simulink model "Gesha1slmodif"  (R2022b)
settings: Solver=VariableStepAuto  StartTime=0.0  StopTime=10.0  RelTol=1e-3
undefined symbols (not defined in the file or in its folder): DiscIntNeverNeededParam
libraries: simulink x13, rllib x1
settings Model: Creator=yonat  LastModifiedBy=Gesha

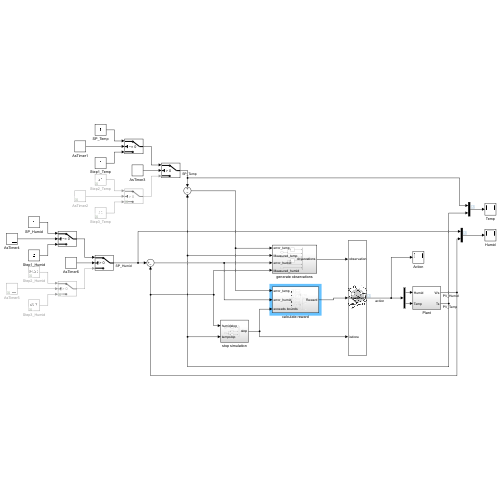
[thumbnail: Simulink's stored preview of the top-level diagram]
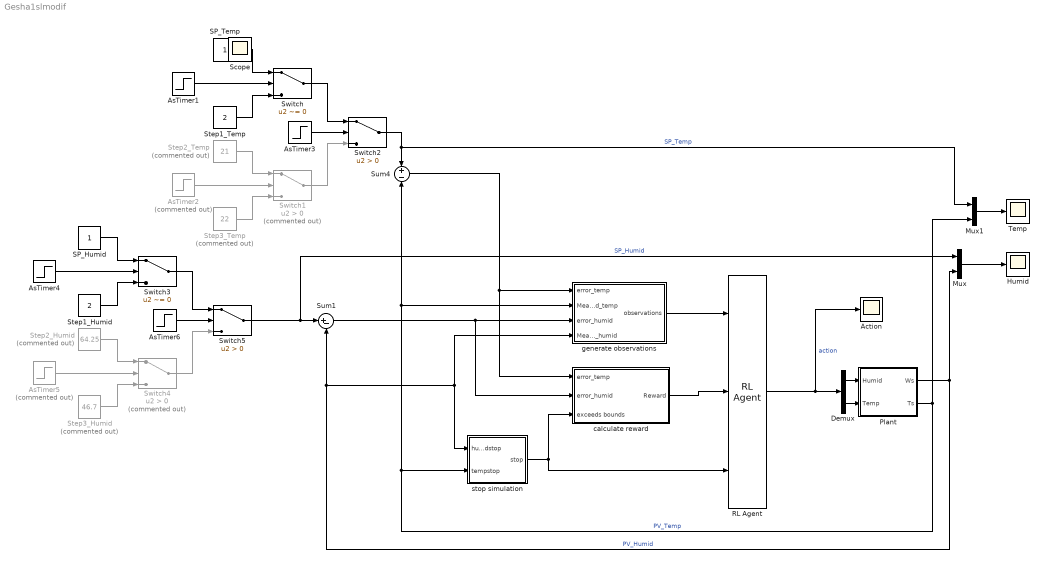
== system Gesha1slmodif ==
  Action : Scope
  AsTimer{1,3..4,6} (4 alike) : Step  Time=5000  Before=1  After=0  SampleTime=0
  AsTimer2 : Step  Commented=on  Time=600  Before=1  After=0  SampleTime=0
  AsTimer5 : Step  Commented=on  Time=600  Before=1  After=0  SampleTime=0
  Demux : Demux  Outputs=2
  Humid : Scope
  Mux : Mux  Inputs=2
  Mux1 : Mux  Inputs=2
  Plant : Subsystem
  RL Agent : rllib/RL Agent  Agent=agent  ExternalActionAsInput=off  ProvideLastAction=off  ProvideCumRwd=off  TreatAsDirectFeedthrough=on  UseStrictObservationDataTypes=off
  SP_Humid : Constant
  SP_Temp : Constant
  Step1_Humid : Constant  Value=2
  Step1_Temp : Constant  Value=2
  Step2_Humid : Constant  Commented=on  Value=64.25
  Step2_Temp : Constant  Commented=on  Value=21
  Step3_Humid : Constant  Commented=on  Value=46.7
  Step3_Temp : Constant  Commented=on  Value=22
  Sum1 : Sum  Inputs=|+-  SaturateOnIntegerOverflow=on
  Sum4 : Sum  Inputs=+-  SaturateOnIntegerOverflow=on
  Switch : Switch  Criteria=u2 ~= 0  Threshold=1  SaturateOnIntegerOverflow=off  InputSameDT=off
  Switch1 : Switch  Commented=on  Criteria=u2 > Threshold  SaturateOnIntegerOverflow=off  InputSameDT=off
  Switch2 : Switch  Criteria=u2 > Threshold  SaturateOnIntegerOverflow=off  InputSameDT=off
  Switch3 : Switch  Criteria=u2 ~= 0  Threshold=1  SaturateOnIntegerOverflow=off  InputSameDT=off
  Switch4 : Switch  Commented=on  Criteria=u2 > Threshold  SaturateOnIntegerOverflow=off  InputSameDT=off
  Switch5 : Switch  Criteria=u2 > Threshold  SaturateOnIntegerOverflow=off  InputSameDT=off
  Temp : Scope
  calculate reward : Subsystem
  generate observations : Subsystem
  stop simulation : Subsystem
  Scope : Scope
  wires:
  stop simulation/1(stop) -> RL Agent/3, calculate reward/3(exceeds bounds)
  Plant/2(Ts) -> Mux1/2, generate observations/2(Measured_temp), Sum4/2, stop simulation/2(tempstop)  "PV_Temp"
  Sum4/1 -> calculate reward/1(error_temp), generate observations/1(error_temp)
  Plant/1(Ws) -> Mux/2, generate observations/4(Measured_humid), stop simulation/1(humidstop), Sum1/2  "PV_Humid"
  Sum1/1 -> calculate reward/2(error_humid), generate observations/3(error_humid)
  RL Agent/1 -> Action/1, Demux/1  "action"
  generate observations/1(observations) -> RL Agent/1
  Demux/2 -> Plant/2(Temp)
  Demux/1 -> Plant/1(Humid)
  SP_Temp/1 -> Switch/1
  AsTimer1/1 -> Switch/2
  Step3_Temp/1 -> Switch1/3
  Step1_Temp/1 -> Switch/3
  Switch/1 -> Switch2/1
  Switch1/1 -> Switch2/3
  AsTimer3/1 -> Switch2/2
  Step2_Temp/1 -> Switch1/1
  AsTimer2/1 -> Switch1/2
  Switch2/1 -> Mux1/1, Sum4/1  "SP_Temp"
  AsTimer6/1 -> Switch5/2
  Step2_Humid/1 -> Switch4/1
  AsTimer5/1 -> Switch4/2
  Switch4/1 -> Switch5/3
  Step3_Humid/1 -> Switch4/3
  AsTimer4/1 -> Switch3/2
  Switch3/1 -> Switch5/1
  Step1_Humid/1 -> Switch3/3
  SP_Humid/1 -> Switch3/1
  Switch5/1 -> Mux/1, Sum1/1  "SP_Humid"
  calculate reward/1(Reward) -> RL Agent/2
  Mux/1 -> Humid/1
  Mux1/1 -> Temp/1

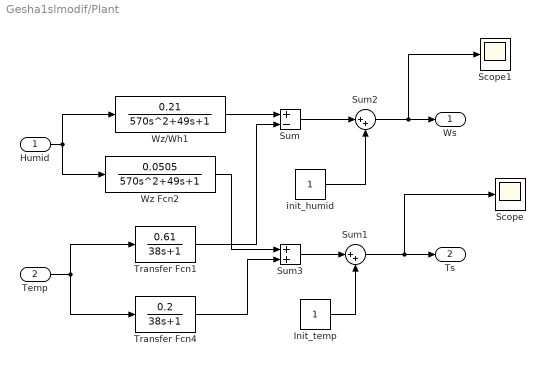
== system Gesha1slmodif/Plant ==
  Humid : Inport
  Temp : Inport  Port=2
  Init_temp : Constant
  Scope : Scope
  Scope1 : Scope
  Sum : Sum  Inputs=+-
  Sum1 : Sum  Inputs=|++
  Sum2 : Sum  Inputs=|++
  Sum3 : Sum
  Transfer Fcn1 : TransferFcn  Numerator=[0.61]  Denominator=[38 1]
  Transfer Fcn4 : TransferFcn  Numerator=[0.2]  Denominator=[38 1]
  Wz Fcn2 : TransferFcn  Numerator=[0.0505]  Denominator=[570 49 1]
  Wz/Wh1 : TransferFcn  Numerator=[0.21]  Denominator=[570 49 1]
  init_humid : Constant
  Ws : Outport
  Ts : Outport  Port=2
  wires:
  Wz Fcn2/1 -> Sum3/1
  Humid/1 -> Wz/Wh1/1, Wz Fcn2/1
  Temp/1 -> Transfer Fcn1/1, Transfer Fcn4/1
  Transfer Fcn1/1 -> Sum/2
  Wz/Wh1/1 -> Sum/1
  Transfer Fcn4/1 -> Sum3/2
  Sum/1 -> Sum2/1
  Sum3/1 -> Sum1/1
  Sum1/1 -> Scope/1, Ts/1
  Sum2/1 -> Scope1/1, Ws/1
  Init_temp/1 -> Sum1/2
  init_humid/1 -> Sum2/2

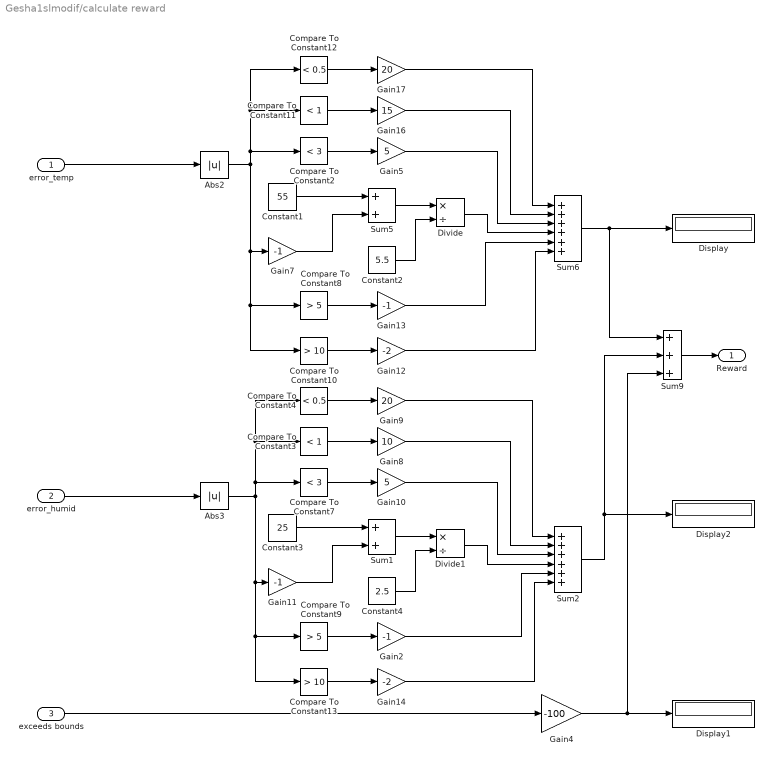
== system Gesha1slmodif/calculate reward ==
  error_temp : Inport
  error_humid : Inport  Port=2
  exceeds bounds : Inport  Port=3
  Abs2 : Abs  SaturateOnIntegerOverflow=off
  Abs3 : Abs  SaturateOnIntegerOverflow=off
  Compare To Constant10 : simulink/Logic and Bit Operations/Compare To Constant  relop=>  const=10  OutDataTypeStr=boolean
  Compare To Constant11 : simulink/Logic and Bit Operations/Compare To Constant  relop=<  const=1  OutDataTypeStr=boolean
  Compare To Constant12 : simulink/Logic and Bit Operations/Compare To Constant  relop=<  const=0.5  OutDataTypeStr=boolean
  Compare To Constant13 : simulink/Logic and Bit Operations/Compare To Constant  relop=>  const=10  OutDataTypeStr=boolean
  Compare To Constant2 : simulink/Logic and Bit Operations/Compare To Constant  relop=<  const=3  OutDataTypeStr=boolean
  Compare To Constant3 : simulink/Logic and Bit Operations/Compare To Constant  relop=<  const=1  OutDataTypeStr=boolean
  Compare To Constant4 : simulink/Logic and Bit Operations/Compare To Constant  relop=<  const=0.5  OutDataTypeStr=boolean
  Compare To Constant7 : simulink/Logic and Bit Operations/Compare To Constant  relop=<  const=3  OutDataTypeStr=boolean
  Compare To Constant8 : simulink/Logic and Bit Operations/Compare To Constant  relop=>  const=5  OutDataTypeStr=boolean
  Compare To Constant9 : simulink/Logic and Bit Operations/Compare To Constant  relop=>  const=5  OutDataTypeStr=boolean
  Constant1 : Constant  Value=55
  Constant2 : Constant  Value=5.5
  Constant3 : Constant  Value=25
  Constant4 : Constant  Value=2.5
  Display : Display
  Display1 : Display
  Display2 : Display
  Divide : Product  Inputs=*/
  Divide1 : Product  Inputs=*/
  Gain10 : Gain  Gain=5
  Gain{2,7,11,13} (4 alike) : Gain  Gain=-1
  Gain12 : Gain  Gain=-2
  Gain14 : Gain  Gain=-2
  Gain16 : Gain  Gain=15
  Gain17 : Gain  Gain=20
  Gain4 : Gain  Gain=-100
  Gain5 : Gain  Gain=5
  Gain8 : Gain  Gain=10
  Gain9 : Gain  Gain=20
  Sum1 : Sum
  Sum2 : Sum  Inputs=6
  Sum5 : Sum
  Sum6 : Sum  Inputs=6
  Sum9 : Sum  Inputs=+++
  Reward : Outport
  wires:
  Sum2/1 -> Display2/1, Sum9/2
  error_temp/1 -> Abs2/1
  Gain7/1 -> Sum5/2
  Compare To Constant7/1 -> Gain10/1
  Divide/1 -> Sum6/4
  Compare To Constant8/1 -> Gain13/1
  Compare To Constant4/1 -> Gain9/1
  Constant4/1 -> Divide1/2
  Gain9/1 -> Sum2/1
  Abs3/1 -> Gain11/1, Compare To Constant13/1, Compare To Constant9/1, Compare To Constant4/1, Compare To Constant3/1, Compare To Constant7/1
  Compare To Constant13/1 -> Gain14/1
  Gain13/1 -> Sum6/5
  Sum9/1 -> Reward/1
  Divide1/1 -> Sum2/4
  Constant3/1 -> Sum1/1
  Constant2/1 -> Divide/2
  Gain8/1 -> Sum2/2
  Gain12/1 -> Sum6/6
  Compare To Constant11/1 -> Gain16/1
  Compare To Constant9/1 -> Gain2/1
  Compare To Constant3/1 -> Gain8/1
  error_humid/1 -> Abs3/1
  Gain11/1 -> Sum1/2
  Sum5/1 -> Divide/1
  Sum1/1 -> Divide1/1
  Gain4/1 -> Display1/1, Sum9/3
  exceeds bounds/1 -> Gain4/1
  Compare To Constant10/1 -> Gain12/1
  Abs2/1 -> Compare To Constant2/1, Compare To Constant11/1, Compare To Constant12/1, Compare To Constant10/1, Compare To Constant8/1, Gain7/1
  Compare To Constant12/1 -> Gain17/1
  Compare To Constant2/1 -> Gain5/1
  Gain14/1 -> Sum2/6
  Gain2/1 -> Sum2/5
  Gain10/1 -> Sum2/3
  Sum6/1 -> Sum9/1, Display/1
  Gain16/1 -> Sum6/2
  Gain5/1 -> Sum6/3
  Gain17/1 -> Sum6/1
  Constant1/1 -> Sum5/1

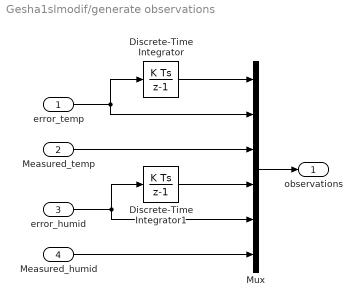
== system Gesha1slmodif/generate observations ==
  error_temp : Inport
  Measured_temp : Inport  Port=2
  error_humid : Inport  Port=3
  Measured_humid : Inport  Port=4
  Discrete-Time Integrator : DiscreteIntegrator  SampleTime=1.0  ICPrevOutput=DiscIntNeverNeededParam  ICPrevScaledInput=DiscIntNeverNeededParam
  Discrete-Time Integrator1 : DiscreteIntegrator  SampleTime=1.0  ICPrevOutput=DiscIntNeverNeededParam  ICPrevScaledInput=DiscIntNeverNeededParam
  Mux : Mux  Inputs=6
  observations : Outport  VectorParamsAs1DForOutWhenUnconnected=off
  wires:
  error_temp/1 -> Discrete-Time Integrator/1, Mux/2
  error_humid/1 -> Mux/5, Discrete-Time Integrator1/1
  Discrete-Time Integrator1/1 -> Mux/4
  Discrete-Time Integrator/1 -> Mux/1
  Measured_temp/1 -> Mux/3
  Measured_humid/1 -> Mux/6
  Mux/1 -> observations/1

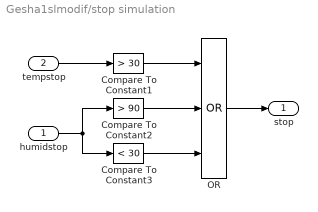
== system Gesha1slmodif/stop simulation ==
  humidstop : Inport
  tempstop : Inport  Port=2
  Compare To Constant1 : simulink/Logic and Bit Operations/Compare To Constant  relop=>  const=30  OutDataTypeStr=boolean
  Compare To Constant2 : simulink/Logic and Bit Operations/Compare To Constant  relop=>  const=90  OutDataTypeStr=boolean
  Compare To Constant3 : simulink/Logic and Bit Operations/Compare To Constant  relop=<  const=30  OutDataTypeStr=boolean
  OR : Logic  Operator=OR  Inputs=3  IconShape=distinctive  AllPortsSameDT=off  OutDataTypeStr=boolean
  stop : Outport  VectorParamsAs1DForOutWhenUnconnected=off
  wires:
  tempstop/1 -> Compare To Constant1/1
  humidstop/1 -> Compare To Constant2/1, Compare To Constant3/1
  Compare To Constant1/1 -> OR/1
  Compare To Constant3/1 -> OR/3
  OR/1 -> stop/1
  Compare To Constant2/1 -> OR/2
